simulink model "control_cascada"  (R2023a)
settings: Solver=FixedStepAuto  StartTime=0.0  StopTime=10.0  FixedStep=0.030  RelTol=1e-3
values from neighbouring files (symbols this model uses):
  a = 0.2    [control_posicion.m]
undefined symbols (not defined in the file or in its folder): out
libraries: slpidlib x2
settings Model: Creator=oem  LastModifiedBy=oem

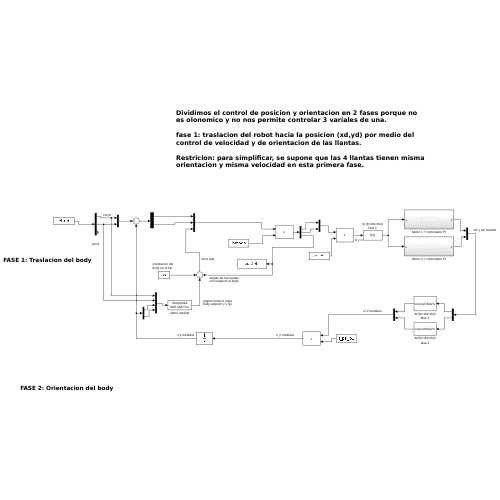
[thumbnail: Simulink's stored preview of the top-level diagram]
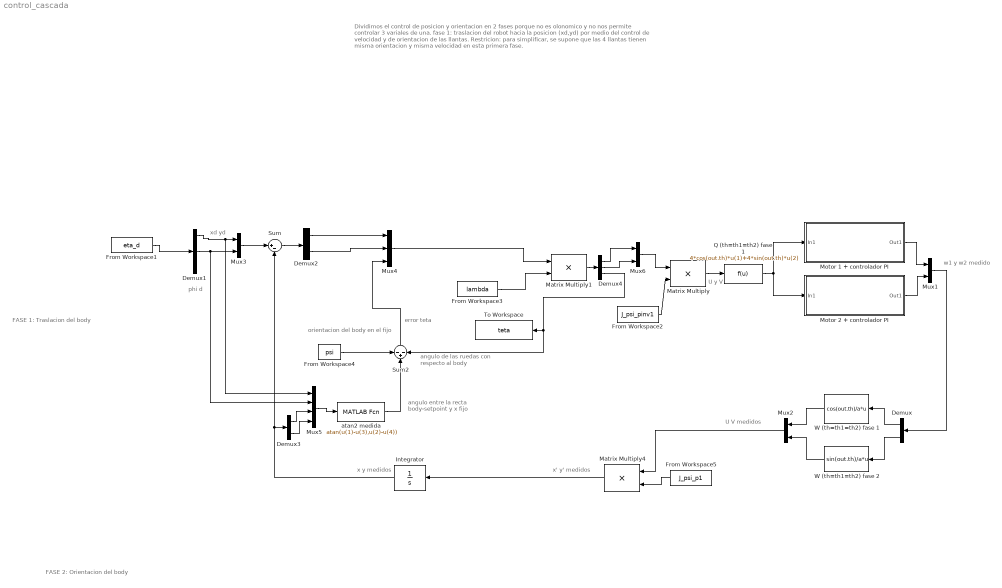
== system control_cascada ==
  note: angulo de las ruedas con respecto al body
  note: orientacion del body en el fijo
  note: FASE 1: Traslacion del body
  note: Dividimos el control de posicion y orientacion en 2 fases porque no es olonomico y no nos permite controlar 3 variales de una.
      |
      | fase 1: traslacion del robot hacia la posicion (xd,yd) por medio del control de velocidad y de orientacion de las llantas.
      |
      | Restricion: para simplificar, se supone que las 4 llantas tienen misma orientacion y misma velocidad en esta primera fase.
  note: U y V
  note: error teta
  note: phi d
  note: xd yd
  note: x y medidos
  note: x' y' medidos
  note: w1 y w2 medido
  note: U V medidos
  note: FASE 2: Orientacion del body
  note: angulo entre la recta body-setpoint y x fijo
  Demux : Demux  Outputs=2
  Demux1 : Demux  Outputs=3
  Demux2 : Demux  Outputs=2
  Demux3 : Demux  Outputs=2
  Demux4 : Demux  Outputs=3
  From Workspace1 : FromWorkspace  VariableName=eta_d
  From Workspace2 : FromWorkspace  VariableName=J_psi_pinv1
  From Workspace3 : FromWorkspace  VariableName=lambda
  From Workspace4 : FromWorkspace  VariableName=psi
  From Workspace5 : FromWorkspace  VariableName=J_psi_p1
  Integrator : Integrator
  Matrix Multiply : Product
  Matrix Multiply1 : Product
  Matrix Multiply4 : Product
  Motor 1 + controlador PI : Subsystem
  Motor 2 + controlador PI : Subsystem
  Mux{1..3,6} (4 alike) : Mux  Inputs=2
  Mux4 : Mux  Inputs=3
  Mux5 : Mux
  Q (th=th1=th2) fase 1 : Fcn  Expr=4*cos(out.th)*u(1)+4*sin(out.th)*u(2)
  Sum : Sum  Inputs=|+-
  Sum2 : Sum  Inputs=-+-
  To Workspace : ToWorkspace  VariableName=teta  SaveFormat=Timeseries  SampleTime=-1
  W (th=th1=th2) fase 1 : Fcn  Expr=cos(out.th)/a*u
  W (th=th1=th2) fase 2 : Fcn  Expr=sin(out.th)/a*u
  atan2 medida : MATLABFcn  MATLABFcn=atan(u(1)-u(3),u(2)-u(4))
  wires:
  Integrator/1 -> Sum/2, Demux3/1
  From Workspace2/1 -> Matrix Multiply/2
  Demux4/3 -> Sum2/3, To Workspace/1
  From Workspace3/1 -> Matrix Multiply1/2
  Motor 1 + controlador PI/1(Out1) -> Mux1/1
  Motor 2 + controlador PI/1(Out1) -> Mux1/2
  Matrix Multiply4/1 -> Integrator/1
  From Workspace5/1 -> Matrix Multiply4/2
  Mux4/1 -> Matrix Multiply1/1
  Matrix Multiply/1 -> Q (th=th1=th2) fase 1/1
  Q (th=th1=th2) fase 1/1 -> Motor 2 + controlador PI/1(In1), Motor 1 + controlador PI/1(In1)
  W (th=th1=th2) fase 1/1 -> Mux2/1
  W (th=th1=th2) fase 2/1 -> Mux2/2
  Mux2/1 -> Matrix Multiply4/1
  Demux/2 -> W (th=th1=th2) fase 2/1
  Demux/1 -> W (th=th1=th2) fase 1/1
  Mux1/1 -> Demux/1
  From Workspace1/1 -> Demux1/1
  Demux1/1 -> Mux5/1, Mux3/1
  Demux1/2 -> Mux3/2, Mux5/2
  Mux3/1 -> Sum/1
  Demux3/2 -> Mux5/4
  Demux3/1 -> Mux5/3
  Mux5/1 -> atan2 medida/1
  atan2 medida/1 -> Sum2/2
  Sum2/1 -> Mux4/3
  Demux2/2 -> Mux4/2
  Demux2/1 -> Mux4/1
  Sum/1 -> Demux2/1
  From Workspace4/1 -> Sum2/1
  Matrix Multiply1/1 -> Demux4/1
  Demux4/2 -> Mux6/2
  Demux4/1 -> Mux6/1
  Mux6/1 -> Matrix Multiply/1

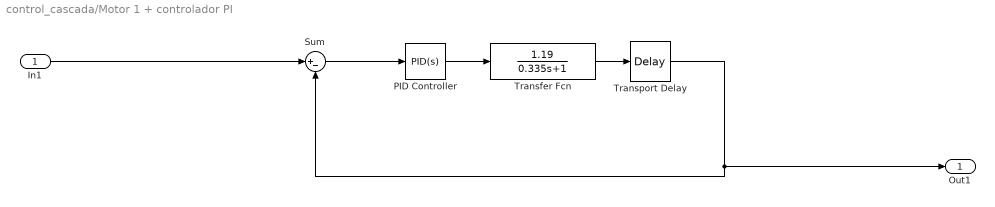
== system control_cascada/Motor 1 + controlador PI ==
  In1 : Inport
  PID Controller : slpidlib/PID Controller  Controller=PID  Form=Parallel  TimeDomain=Continuous-time  UseExternalTs=off  SampleTime=-1  IntegratorMethod=Forward Euler  FilterMethod=Forward Euler  ControllerParametersSource=internal  P=4  I=4  UseKiTs=off  D=0  N=100  UseFilter=on  TunerSelectOption=Transfer Function Based (PID Tuner App)  InitialConditionSource=internal  InitialConditionForIntegrator=0  InitialConditionForFilter=0  DifferentiatorICPrevScaledInput=0  ExternalReset=none  TrackingMode=off  Kt=1  LimitOutput=off  SatLimitsSource=internal  UpperSaturationLimit=inf  LowerSaturationLimit=-inf  LinearizeAsGain=on  AntiWindupMode=none  Kb=1  LimitIntegrator=off  UpperIntegratorSaturationLimit=inf  LowerIntegratorSaturationLimit=-inf  POutMin=[]  POutMax=[]  IOutMin=[]  IOutMax=[]  DOutMin=[]  DOutMax=[]  NOutMin=[]  NOutMax=[]  SumOutMin=[]  SumOutMax=[]  SaturationOutMin=[]  SaturationOutMax=[]  PParamMin=[]  PParamMax=[]  IParamMin=[]  IParamMax=[]  DParamMin=[]  DParamMax=[]  NParamMin=[]  NParamMax=[]  KbParamMin=[]  KbParamMax=[]  KtParamMin=[]  KtParamMax=[]  KbOutMin=[]  KbOutMax=[]  KtOutMin=[]  KtOutMax=[]  IntegratorOutMin=[]  IntegratorOutMax=[]  FilterOutMin=[]  FilterOutMax=[]  SumI1OutMin=[]  SumI1OutMax=[]  SumI2OutMin=[]  SumI2OutMax=[]  SumI3OutMin=[]  SumI3OutMax=[]  SumI4OutMin=[]  SumI4OutMax=[]  SumDOutMin=[]  SumDOutMax=[]  DifferentiatorOutMin=[]  DifferentiatorOutMax=[]  FilterDiffOutCoefMin=[]  FilterDiffOutCoefMax=[]  ReciprocalOutMin=[]  ReciprocalOutMax=[]  SumDenOutMin=[]  SumDenOutMax=[]  SumNumOutMin=[]  SumNumOutMax=[]  DivideOutMin=[]  DivideOutMax=[]  UdiffTsProdOutMin=[]  UdiffTsProdOutMax=[]  NTsProdOutMin=[]  NTsProdOutMax=[]  UintegralTsProdOutMin=[]  UintegralTsProdOutMax=[]  UngainTsProdOutMin=[]  UngainTsProdOutMax=[]  ClampingZeroOutDataTypeStr=Inherit: Inherit via back propagation  ClampingZeroOutMin=[]  ClampingZeroOutMax=[]  FilterDenConstantOutDataTypeStr=Inherit: Inherit via back propagation  FilterDenConstantOutMin=[]  FilterDenConstantOutMax=[]  PCopyOutDataTypeStr=Inherit: Inherit via back propagation  PCopyOutMin=[]  PCopyOutMax=[]  NCopyOutDataTypeStr=Inherit: Inherit via back propagation  NCopyOutMin=[]  NCopyOutMax=[]  IntegratorContinuousStateAttributes=''  IntegratorStateMustResolveToSignalObject=off  IntegratorRTWStateStorageClass=Auto  FilterContinuousStateAttributes=''  FilterStateMustResolveToSignalObject=off  FilterRTWStateStorageClass=Auto  ParallelPVariant=InternalParameters  IdealPVariant=Disabled  IVariant=InternalParameters  DVariant=InternalParameters  IntegratorVariant=Continuous  SatVariant=Disabled  AWVariant=Passthrough  PCopyVariant=Disabled  TRVariant=Disabled  FdbkBlocksVariant=Forward  IdealPFdbkVariant=Disabled  SatFdbkVariant=Disabled  DerivativeFilterVariant=ContFilter  NVariant=InternalParameters  NCopyVariant=Disabled  FilterICVariant=InternalICsFilter  IntegratorICVariant=InternalICs  ExternalResetVariant=Disabled  TRSumVariant=Passthrough  SumFdbkVariant=Disabled  SumVariant=Sum_PID  TsampFilterVariant=InternalTs  TsampNgainVariant=Passthrough  TsampIntegralVariant=Disabled_SignalSpec  ExternalSaturationOutDataTypeStr=Inherit: Same as second input
  Sum : Sum  Inputs=|+-
  Transfer Fcn : TransferFcn  Numerator=[1.19]  Denominator=[0.335 1]
  Transport Delay : TransportDelay  DelayTime=0.01
  Out1 : Outport
  wires:
  In1/1 -> Sum/1
  PID Controller/1 -> Transfer Fcn/1
  Transfer Fcn/1 -> Transport Delay/1
  Sum/1 -> PID Controller/1
  Transport Delay/1 -> Out1/1, Sum/2

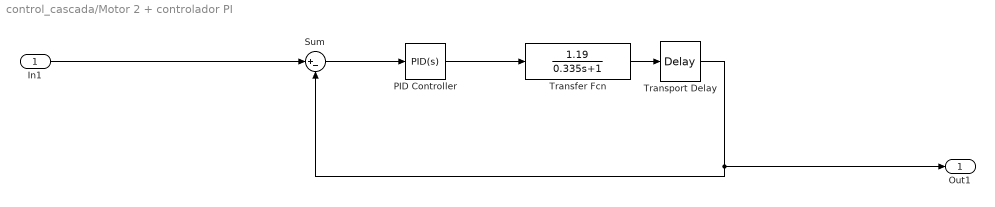
== system control_cascada/Motor 2 + controlador PI ==
  In1 : Inport
  PID Controller : slpidlib/PID Controller  Controller=PID  Form=Parallel  TimeDomain=Continuous-time  UseExternalTs=off  SampleTime=-1  IntegratorMethod=Forward Euler  FilterMethod=Forward Euler  ControllerParametersSource=internal  P=4  I=4  UseKiTs=off  D=0  N=100  UseFilter=on  TunerSelectOption=Transfer Function Based (PID Tuner App)  InitialConditionSource=internal  InitialConditionForIntegrator=0  InitialConditionForFilter=0  DifferentiatorICPrevScaledInput=0  ExternalReset=none  TrackingMode=off  Kt=1  LimitOutput=off  SatLimitsSource=internal  UpperSaturationLimit=inf  LowerSaturationLimit=-inf  LinearizeAsGain=on  AntiWindupMode=none  Kb=1  LimitIntegrator=off  UpperIntegratorSaturationLimit=inf  LowerIntegratorSaturationLimit=-inf  POutMin=[]  POutMax=[]  IOutMin=[]  IOutMax=[]  DOutMin=[]  DOutMax=[]  NOutMin=[]  NOutMax=[]  SumOutMin=[]  SumOutMax=[]  SaturationOutMin=[]  SaturationOutMax=[]  PParamMin=[]  PParamMax=[]  IParamMin=[]  IParamMax=[]  DParamMin=[]  DParamMax=[]  NParamMin=[]  NParamMax=[]  KbParamMin=[]  KbParamMax=[]  KtParamMin=[]  KtParamMax=[]  KbOutMin=[]  KbOutMax=[]  KtOutMin=[]  KtOutMax=[]  IntegratorOutMin=[]  IntegratorOutMax=[]  FilterOutMin=[]  FilterOutMax=[]  SumI1OutMin=[]  SumI1OutMax=[]  SumI2OutMin=[]  SumI2OutMax=[]  SumI3OutMin=[]  SumI3OutMax=[]  SumI4OutMin=[]  SumI4OutMax=[]  SumDOutMin=[]  SumDOutMax=[]  DifferentiatorOutMin=[]  DifferentiatorOutMax=[]  FilterDiffOutCoefMin=[]  FilterDiffOutCoefMax=[]  ReciprocalOutMin=[]  ReciprocalOutMax=[]  SumDenOutMin=[]  SumDenOutMax=[]  SumNumOutMin=[]  SumNumOutMax=[]  DivideOutMin=[]  DivideOutMax=[]  UdiffTsProdOutMin=[]  UdiffTsProdOutMax=[]  NTsProdOutMin=[]  NTsProdOutMax=[]  UintegralTsProdOutMin=[]  UintegralTsProdOutMax=[]  UngainTsProdOutMin=[]  UngainTsProdOutMax=[]  ClampingZeroOutDataTypeStr=Inherit: Inherit via back propagation  ClampingZeroOutMin=[]  ClampingZeroOutMax=[]  FilterDenConstantOutDataTypeStr=Inherit: Inherit via back propagation  FilterDenConstantOutMin=[]  FilterDenConstantOutMax=[]  PCopyOutDataTypeStr=Inherit: Inherit via back propagation  PCopyOutMin=[]  PCopyOutMax=[]  NCopyOutDataTypeStr=Inherit: Inherit via back propagation  NCopyOutMin=[]  NCopyOutMax=[]  IntegratorContinuousStateAttributes=''  IntegratorStateMustResolveToSignalObject=off  IntegratorRTWStateStorageClass=Auto  FilterContinuousStateAttributes=''  FilterStateMustResolveToSignalObject=off  FilterRTWStateStorageClass=Auto  ParallelPVariant=InternalParameters  IdealPVariant=Disabled  IVariant=InternalParameters  DVariant=InternalParameters  IntegratorVariant=Continuous  SatVariant=Disabled  AWVariant=Passthrough  PCopyVariant=Disabled  TRVariant=Disabled  FdbkBlocksVariant=Forward  IdealPFdbkVariant=Disabled  SatFdbkVariant=Disabled  DerivativeFilterVariant=ContFilter  NVariant=InternalParameters  NCopyVariant=Disabled  FilterICVariant=InternalICsFilter  IntegratorICVariant=InternalICs  ExternalResetVariant=Disabled  TRSumVariant=Passthrough  SumFdbkVariant=Disabled  SumVariant=Sum_PID  TsampFilterVariant=InternalTs  TsampNgainVariant=Passthrough  TsampIntegralVariant=Disabled_SignalSpec  ExternalSaturationOutDataTypeStr=Inherit: Same as second input
  Sum : Sum  Inputs=|+-
  Transfer Fcn : TransferFcn  Numerator=[1.19]  Denominator=[0.335 1]
  Transport Delay : TransportDelay  DelayTime=0.01
  Out1 : Outport
  wires:
  In1/1 -> Sum/1
  PID Controller/1 -> Transfer Fcn/1
  Transfer Fcn/1 -> Transport Delay/1
  Sum/1 -> PID Controller/1
  Transport Delay/1 -> Out1/1, Sum/2
